simulink model "sampleModel1470"  (R2023a)
settings: Solver=VariableStepAuto  StartTime=0.0  StopTime=10.0  RelTol=1e-3
libraries: hdlsllib x3, simulink x3
settings Model: Creator=user1  LastModifiedBy=user1

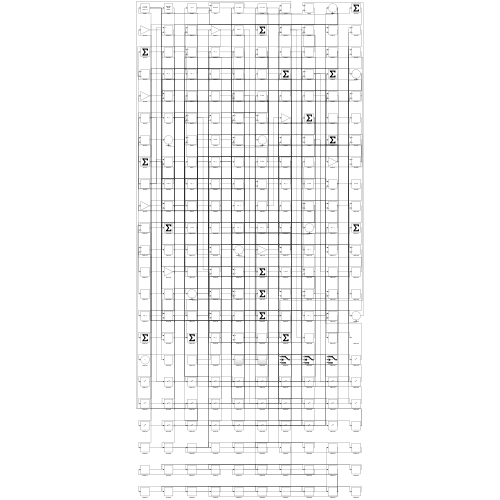
[thumbnail: Simulink's stored preview of the top-level diagram]
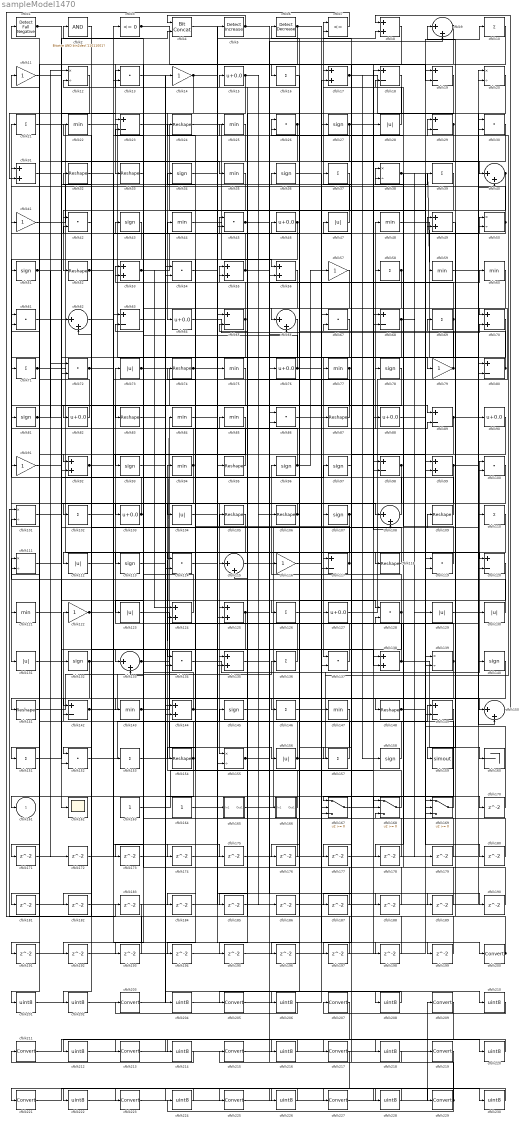
== system sampleModel1470 ==
  cfblk1 : hdlsllib/Logic and Bit Operations/Detect Fall Negative  vinit=0  OutDataTypeStr=boolean
  cfblk{10,16,21,37,39,58,69,71,102,110,126,136,146,151,153,157} (16 alike) : Sum  Inputs=+
  cfblk{13,26,30,42,45,54,61,67,72,86,100,114,119,128,134,137,152} (17 alike) : DotProduct  OutDataTypeStr=Inherit: Inherit via internal rule
  cfblk{12,20,38,50,101,111,139,155} (8 alike) : Product  Inputs=*/  RndMeth=Zero  SaturateOnIntegerOverflow=on
  cfblk{15,46,64,76,82,88,90,103,127} (9 alike) : Bias  Bias=0.0  SaturateOnIntegerOverflow=off
  cfblk{28,47,73,104,112,123,129..131,156} (10 alike) : Abs  SaturateOnIntegerOverflow=off
  cfblk{24,32..33,52,74,83,87,95,105..106,109,118,141,148,154} (15 alike) : Reshape
  cfblk{27,34,36,43,51,78,81,93,96..97,107,113,132,140,145,158} (16 alike) : Signum
  cfblk{9,40,62,66,108,115,133,150} (8 alike) : Sum  Inputs=|++
  cfblk{11,14,41,57,79,91,116,122} (8 alike) : Gain
  cfblk{18..19,23,29,63,65,68,80,89,98,117,120,142,149} (14 alike) : Sum  Inputs=+-
  cfblk{22,25,35,44,48,59..60,75,77,84..85,94,121,143,147} (15 alike) : MinMax
  cfblk{8,17,31,49,53,55..56,70,92,99,124..125,135,138,144} (15 alike) : Sum
  cfblk159 : ToWorkspace  VariableName=simout  SaveFormat=Timeseries  SampleTime=-1
  cfblk160 : Terminator
  cfblk162 : Scope
  cfblk163 : Constant  SampleTime=-1
  cfblk164 : Constant  SampleTime=-1
  cfblk165 : Subsystem
      settings: LibrarySourceBlock=|
      | hdlsllib/Ports &
      | Subsystems/Subsystem
  cfblk166 : Subsystem
      settings: LibrarySourceBlock=|
      | hdlsllib/Ports &
      | Subsystems/Subsystem
  cfblk167 : Switch  SaturateOnIntegerOverflow=off  InputSameDT=off
  cfblk168 : Switch  SaturateOnIntegerOverflow=off  InputSameDT=off
  cfblk169 : Switch  SaturateOnIntegerOverflow=off  InputSameDT=off
  cfblk{170..199} (30 alike) : Delay  SampleTime=1
  cfblk2 : simulink/Logic and Bit Operations/Bitwise Operator  logicop=AND  UseBitMask=on  BitMask=bin2dec('11011001')  BitMaskRealWorld=Stored Integer
      settings: LibrarySourceBlock=|
      | hdlsllib/Logic and Bit
      | Operations/Bitwise
      | Operator
  cfblk{200,203,205,207,209,211,213,215,217,219,221,223,225,227,229} (15 alike) : DataTypeConversion  SaturateOnIntegerOverflow=off  RndMeth=Floor
  cfblk{201..202,204,206,208,210,212,214,216,218,220,222,224,226,228,230} (16 alike) : DataTypeConversion  OutDataTypeStr=uint8  SaturateOnIntegerOverflow=off  RndMeth=Floor
  cfblk3 : hdlsllib/Logic and Bit Operations/Compare To Zero  relop=<=  OutDataTypeStr=boolean
  cfblk4 : hdlsllib/Logic and Bit Operations/Bit Concat  numInputs=2
  cfblk5 : simulink/Logic and Bit Operations/Detect Increase  vinit=0.0  OutDataTypeStr=boolean
      settings: LibrarySourceBlock=|
      | hdlsllib/Logic and Bit
      | Operations/Detect
      | Increase
  cfblk6 : simulink/Logic and Bit Operations/Detect Decrease  vinit=0.0  OutDataTypeStr=boolean
      settings: LibrarySourceBlock=|
      | hdlsllib/Logic and Bit
      | Operations/Detect
      | Decrease
  cfblk7 : RelationalOperator  Operator=<=  OutDataTypeStr=boolean  InputSameDT=off
  cfblk161 : Outport  VectorParamsAs1DForOutWhenUnconnected=off
  wires:
  cfblk70/1 -> cfblk137/1
  cfblk127/1 -> cfblk70/1
  cfblk22/1 -> cfblk79/1
  cfblk134/1 -> cfblk100/1
  cfblk158/1 -> cfblk122/1
  cfblk33/1 -> cfblk2/1
  cfblk37/1 -> cfblk137/2
  cfblk146/1 -> cfblk29/1
  cfblk165/1(Out1) -> cfblk109/1
  cfblk81/1 -> cfblk12/1, cfblk138/2, cfblk72/1
  cfblk103/1 -> cfblk21/1, cfblk193/1
  cfblk46/1 -> cfblk131/1, cfblk134/1
  cfblk86/1 -> cfblk87/1
  cfblk9/1 -> cfblk16/1, cfblk142/1, cfblk197/1
  cfblk15/1 -> cfblk64/1, cfblk106/1
  cfblk136/1 -> cfblk73/1
  cfblk21/1 -> cfblk117/1
  cfblk133/1 -> cfblk84/1, cfblk30/2
  cfblk151/1 -> cfblk62/1
  cfblk121/1 -> cfblk97/1
  cfblk100/1 -> cfblk121/1
  cfblk143/1 -> cfblk48/1, cfblk148/1
  cfblk98/1 -> cfblk155/1, cfblk135/2
  cfblk128/1 -> cfblk96/1, cfblk154/1
  cfblk166/1(Out1) -> cfblk94/1
  cfblk68/1 -> cfblk133/1, cfblk129/1, cfblk134/2
  cfblk8/1 -> cfblk33/1
  cfblk2/1 -> cfblk92/1
  cfblk64/1 -> cfblk70/2
  cfblk24/1 -> cfblk56/1
  cfblk47/1 -> cfblk7/1
  cfblk40/1 -> cfblk52/1, cfblk157/1
  cfblk71/1 -> cfblk89/1, cfblk114/2
  cfblk73/1 -> cfblk119/1, cfblk29/2
  cfblk79/1 -> cfblk12/2, cfblk38/2
  cfblk106/1 -> cfblk46/1, cfblk104/1
  cfblk29/1 -> cfblk123/1, cfblk152/1
  cfblk113/1 -> cfblk14/1
  cfblk78/1 -> cfblk146/1
  cfblk117/1 -> cfblk85/1, cfblk34/1, cfblk55/2
  cfblk1/1 -> cfblk35/1, cfblk126/1, cfblk86/2
  cfblk61/1 -> cfblk162/1
  cfblk49/1 -> cfblk159/1
  cfblk50/1 -> cfblk31/1, cfblk49/2
  cfblk169/1 -> cfblk17/1
  cfblk25/1 -> cfblk161/1
  cfblk138/1 -> cfblk160/1, cfblk67/2
  cfblk69/1 -> cfblk6/1, cfblk55/1, cfblk113/1
  cfblk88/1 -> cfblk10/1
  cfblk11/1 -> cfblk23/1
  cfblk96/1 -> cfblk51/1, cfblk57/1
  cfblk144/1 -> cfblk91/1, cfblk190/1
  cfblk95/1 -> cfblk61/1
  cfblk149/1 -> cfblk167/1
  cfblk28/1 -> cfblk7/2
  cfblk153/1 -> cfblk149/1
  cfblk129/1 -> cfblk30/1
  cfblk109/1 -> cfblk32/1
  cfblk74/1 -> cfblk169/2, cfblk120/2, cfblk170/1
  cfblk66/1 -> cfblk114/1
  cfblk43/1 -> cfblk82/1
  cfblk107/1 -> cfblk37/1, cfblk194/1
  cfblk67/1 -> cfblk93/1
  cfblk108/1 -> cfblk43/1
  cfblk163/1 -> cfblk28/1
  cfblk94/1 -> cfblk13/1, cfblk141/1
  cfblk65/1 -> cfblk53/1, cfblk72/2
  cfblk152/1 -> cfblk145/1
  cfblk139/1 -> cfblk124/2, cfblk191/1
  cfblk89/1 -> cfblk98/2, cfblk9/1, cfblk150/2
  cfblk115/1 -> cfblk116/1
  cfblk57/1 -> cfblk117/2
  cfblk92/1 -> cfblk44/1, cfblk39/1, cfblk174/1
  cfblk77/1 -> cfblk81/1, cfblk185/1
  cfblk4/1 -> cfblk75/1
  cfblk123/1 -> cfblk156/1
  cfblk150/1 -> cfblk8/1
  cfblk35/1 -> cfblk102/1
  cfblk122/1 -> cfblk78/1, cfblk25/1
  cfblk82/1 -> cfblk11/1
  cfblk23/1 -> cfblk139/1
  cfblk84/1 -> cfblk50/1
  cfblk58/1 -> cfblk107/1, cfblk143/1
  cfblk167/1 -> cfblk89/2
  cfblk44/1 -> cfblk56/2
  cfblk10/1 -> cfblk83/1
  cfblk19/1 -> cfblk115/1
  cfblk125/1 -> cfblk76/1, cfblk192/1
  cfblk27/1 -> cfblk88/1, cfblk152/2
  cfblk156/1 -> cfblk99/1, cfblk111/2, cfblk101/2
  cfblk3/1 -> cfblk166/1(In1), cfblk108/2
  cfblk30/1 -> cfblk77/1
  cfblk155/1 -> cfblk65/2, cfblk9/2
  cfblk42/1 -> cfblk22/1
  cfblk85/1 -> cfblk151/1
  cfblk6/1 -> cfblk40/1, cfblk71/1
  cfblk114/1 -> cfblk127/1
  cfblk83/1 -> cfblk168/2
  cfblk31/1 -> cfblk132/1
  cfblk102/1 -> cfblk3/1
  cfblk17/1 -> cfblk80/1, cfblk158/1
  cfblk80/1 -> cfblk18/2, cfblk45/1
  cfblk105/1 -> cfblk112/1
  cfblk20/1 -> cfblk100/2
  cfblk154/1 -> cfblk142/2, cfblk181/1
  cfblk76/1 -> cfblk60/1, cfblk23/2
  cfblk104/1 -> cfblk8/2
  cfblk145/1 -> cfblk58/1
  cfblk13/1 -> cfblk119/2
  cfblk52/1 -> cfblk153/1, cfblk108/1, cfblk125/2
  cfblk60/1 -> cfblk144/2
  cfblk130/1 -> cfblk111/1
  cfblk168/1 -> cfblk74/1
  cfblk51/1 -> cfblk4/2, cfblk172/1
  cfblk87/1 -> cfblk15/1
  cfblk148/1 -> cfblk139/2, cfblk130/1
  cfblk39/1 -> cfblk66/1
  cfblk157/1 -> cfblk61/2
  cfblk164/1 -> cfblk165/1(In1)
  cfblk34/1 -> cfblk118/1
  cfblk53/1 -> cfblk5/1, cfblk124/1
  cfblk32/1 -> cfblk99/2
  cfblk26/1 -> cfblk45/2, cfblk201/1
  cfblk41/1 -> cfblk38/1
  cfblk119/1 -> cfblk26/1
  cfblk93/1 -> cfblk128/1
  cfblk12/1 -> cfblk31/2
  cfblk14/1 -> cfblk42/1, cfblk150/1
  cfblk72/1 -> cfblk63/1, cfblk50/2
  cfblk48/1 -> cfblk140/1
  cfblk132/1 -> cfblk49/1, cfblk171/1
  cfblk45/1 -> cfblk66/2, cfblk186/1
  cfblk137/1 -> cfblk24/1
  cfblk99/1 -> cfblk90/1, cfblk135/1
  cfblk118/1 -> cfblk62/2
  cfblk124/1 -> cfblk63/2
  cfblk54/1 -> cfblk200/1
  cfblk101/1 -> cfblk103/1
  cfblk111/1 -> cfblk125/1
  cfblk5/1 -> cfblk19/2, cfblk4/1
  cfblk75/1 -> cfblk92/2
  cfblk141/1 -> cfblk136/1
  cfblk38/1 -> cfblk59/1, cfblk178/1, cfblk179/1, cfblk180/1
  cfblk142/1 -> cfblk95/1, cfblk182/1
  cfblk18/1 -> cfblk68/2
  cfblk55/1 -> cfblk120/1, cfblk41/1
  cfblk116/1 -> cfblk27/1
  cfblk91/1 -> cfblk36/1
  cfblk59/1 -> cfblk20/2
  cfblk131/1 -> cfblk110/1
  cfblk170/1 -> cfblk19/1
  cfblk171/1 -> cfblk17/2
  cfblk172/1 -> cfblk13/2
  cfblk56/1 -> cfblk173/1
  cfblk173/1 -> cfblk18/1
  cfblk174/1 -> cfblk40/2
  cfblk62/1 -> cfblk175/1
  cfblk175/1 -> cfblk138/1
  cfblk120/1 -> cfblk176/1
  cfblk176/1 -> cfblk115/2
  cfblk97/1 -> cfblk177/1
  cfblk177/1 -> cfblk20/1
  cfblk178/1 -> cfblk133/2
  cfblk179/1 -> cfblk128/2
  cfblk180/1 -> cfblk67/1
  cfblk181/1 -> cfblk155/2
  cfblk182/1 -> cfblk167/2
  cfblk7/1 -> cfblk183/1
  cfblk110/1 -> cfblk184/1
  cfblk184/1 -> cfblk68/1
  cfblk185/1 -> cfblk167/3
  cfblk186/1 -> cfblk80/2
  cfblk90/1 -> cfblk187/1
  cfblk187/1 -> cfblk53/2
  cfblk135/1 -> cfblk188/1
  cfblk188/1 -> cfblk65/1
  cfblk36/1 -> cfblk189/1
  cfblk189/1 -> cfblk144/1
  cfblk190/1 -> cfblk168/3
  cfblk191/1 -> cfblk168/1
  cfblk192/1 -> cfblk169/3
  cfblk193/1 -> cfblk101/1
  cfblk194/1 -> cfblk98/1
  cfblk140/1 -> cfblk195/1
  cfblk195/1 -> cfblk169/1
  cfblk16/1 -> cfblk196/1
  cfblk196/1 -> cfblk149/2
  cfblk197/1 -> cfblk26/2
  cfblk126/1 -> cfblk198/1
  cfblk198/1 -> cfblk1/1
  cfblk112/1 -> cfblk199/1
  cfblk199/1 -> cfblk105/1
  cfblk200/1 -> cfblk42/2, cfblk69/1
  cfblk201/1 -> cfblk54/1
  cfblk183/1 -> cfblk202/1
  cfblk202/1 -> cfblk54/2
  cfblk63/1 -> cfblk204/1
  cfblk204/1 -> cfblk147/1
  cfblk147/1 -> cfblk206/1
  cfblk206/1 -> cfblk203/1
  cfblk203/1 -> cfblk208/1
  cfblk208/1 -> cfblk205/1
  cfblk205/1 -> cfblk210/1
  cfblk210/1 -> cfblk207/1
  cfblk207/1 -> cfblk212/1
  cfblk212/1 -> cfblk209/1
  cfblk209/1 -> cfblk214/1
  cfblk214/1 -> cfblk211/1
  cfblk211/1 -> cfblk216/1
  cfblk216/1 -> cfblk213/1
  cfblk213/1 -> cfblk218/1
  cfblk218/1 -> cfblk215/1
  cfblk215/1 -> cfblk220/1
  cfblk220/1 -> cfblk217/1
  cfblk217/1 -> cfblk222/1
  cfblk222/1 -> cfblk219/1
  cfblk219/1 -> cfblk224/1
  cfblk224/1 -> cfblk221/1
  cfblk221/1 -> cfblk226/1
  cfblk226/1 -> cfblk223/1
  cfblk227/1 -> cfblk229/1
  cfblk223/1 -> cfblk228/1
  cfblk228/1 -> cfblk225/1
  cfblk229/1 -> cfblk47/1, cfblk86/1
  cfblk225/1 -> cfblk230/1
  cfblk230/1 -> cfblk227/1

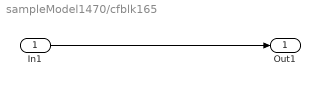
== system sampleModel1470/cfblk165 ==
  In1 : Inport
  Out1 : Outport
  wires:
  In1/1 -> Out1/1

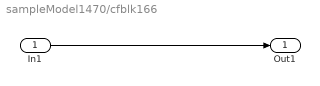
== system sampleModel1470/cfblk166 ==
  In1 : Inport
  Out1 : Outport
  wires:
  In1/1 -> Out1/1
